simulink model "data_exchange_model"  (R2019a)
settings: Solver=VariableStepDiscrete  StartTime=0.0  StopTime=inf  MaxStep=2  RelTol=1e-3
libraries: simulink x1
settings Model: EnablePacing=on  Creator=wuyuanyi  LastModifiedBy=wuyua

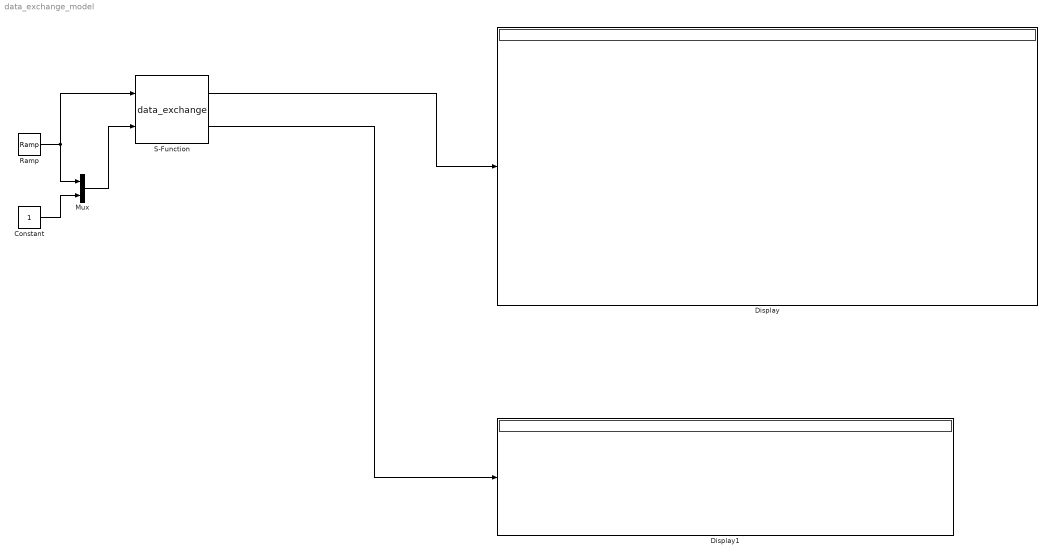
== system data_exchange_model ==
  Constant : Constant
  Display : Display
  Display1 : Display
  Mux : Mux  Inputs=2
  Ramp : simulink/Sources/Ramp  slope=1  start=0  InitialOutput=0
  S-Function : S-Function  FunctionName=data_exchange  SFunctionDeploymentMode=off  EnableBusSupport=off
  wires:
  Mux/1 -> S-Function/2
  Ramp/1 -> Mux/1, S-Function/1
  Constant/1 -> Mux/2
  S-Function/2 -> Display1/1
  S-Function/1 -> Display/1
